simulink model "EKF_UKF_simulation"  (R2022b)
settings: Solver=VariableStepAuto  StartTime=0.0  StopTime=time  RelTol=1e-3
undefined symbols (not defined in the file): dt, R_ublox, sigbuilder_block, X_anchor, Y_anchor
libraries: sharedTrackingLibrary x2
settings Model: Creator=taha  LastModifiedBy=taha

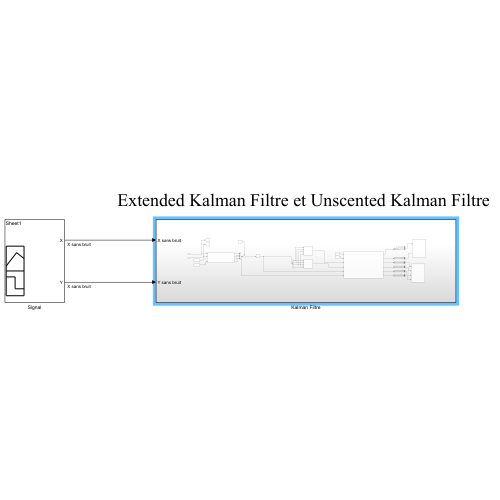
[thumbnail: Simulink's stored preview of the top-level diagram]
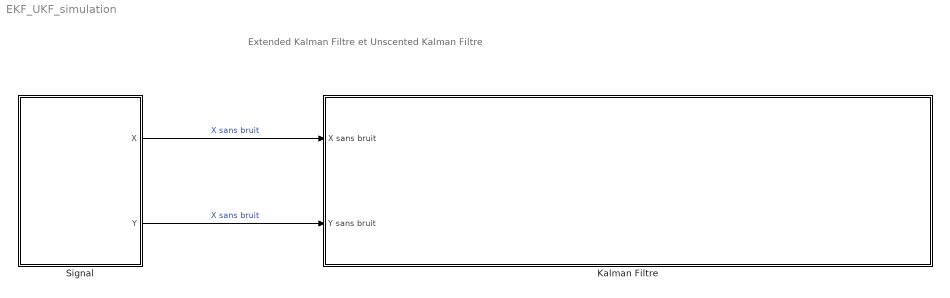
== system EKF_UKF_simulation ==
  note: Extended Kalman Filtre et Unscented Kalman Filtre
  Kalman Filtre : Subsystem
  Signal : Subsystem  Tag=STV Subsys  LoadFcn=sigbuilder_block('load');  StartFcn=sigbuilder_block('start');  StopFcn=sigbuilder_block('stop');  ClipboardFcn=sigbuilder_block('clipboard');  mask(Sigbuilder block){tuvar=[0:10]}
      mask help: Simulink:masks:SigbuilderBlock_MD
      mask init:
      | if ~strcmp(get_param(bdroot(gcbh),'SimulationStatus'),'stopped') tuvar = sigbuilder_block('maskInit'); end
      settings: CopyFcn=sigbuilder_block('copy');  DeleteFcn=sigbuilder_block('delete');  ModelCloseFcn=sigbuilder_block('modelClose');  PreSaveFcn=sigbuilder_block('preSave');  PauseFcn=sigbuilder_block('pause');  ContinueFcn=sigbuilder_block('continue');  NameChangeFcn=sigbuilder_block('namechange');  OpenFcn=sigbuilder_block('open',[6 36 1012.5 441.75 ]);  CloseFcn=sigbuilder_block('close');
      mask Display: plot(0, 0, 100, 100,[2, 2, 32, 32, 2], [68, 8, 8, 68, 68],[32, 2], [38, 38], [32, 19, 2],[53, 60, 44], [32, 17, 17, 2],[16, 16, 31, 31]);txt = getActiveGroup(gcbh);text(2, 100, txt,'verticalAlignment', 'top');
  wires:
  Signal/2(Y) -> Kalman Filtre/2(Y sans bruit)  "X sans bruit"
  Signal/1(X) -> Kalman Filtre/1(X sans bruit)  "X sans bruit"

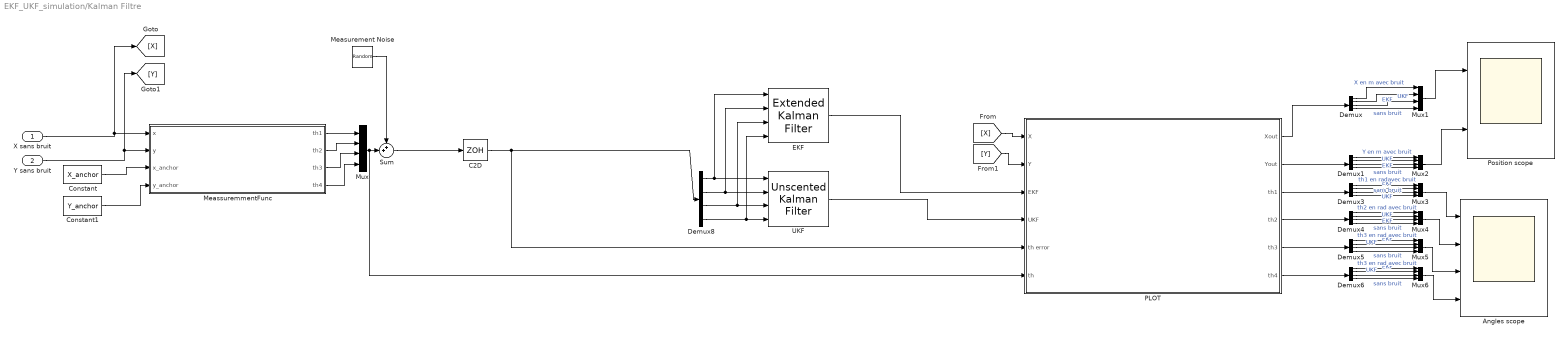
== system EKF_UKF_simulation/Kalman Filtre ==
  X sans bruit : Inport
  Y sans bruit : Inport  Port=2
  Angles scope : Scope  NumInputPorts=4
  C2D : ZeroOrderHold  SampleTime=dt
  Constant : Constant  Value=X_anchor
  Constant1 : Constant  Value=Y_anchor
  Demux{,1,3..6,8} (7 alike) : Demux
  EKF : sharedTrackingLibrary/Extended Kalman Filter  StateTransitionFcn=myStateTransitionFcn  HasStateTransitionJacobianFcn=off  HasAdditiveProcessNoise=Additive  ProcessNoise=Q  HasTimeVaryingProcessNoise=off  HasStateTransitionFcnExtraArgument=0  InitialState=x0  InitialStateCovariance=1  MeasurementFcn1=myMeasurementFcn21  HasMeasurementJacobianFcn1=off  HasMeasurementEnablePort1=off  HasAdditiveMeasurementNoise1=Additive  MeasurementNoise1=sigma_theta0  HasTimeVaryingMeasurementNoise1=off  HasMeasurementFcnExtraArgument1=0  HasMeasurementWrapping1=off  MeasurementFcn2=myMeasurementFcn22  HasMeasurementJacobianFcn2=off  HasMeasurementEnablePort2=off  HasAdditiveMeasurementNoise2=Additive  MeasurementNoise2=sigma_theta0  HasTimeVaryingMeasurementNoise2=off  HasMeasurementFcnExtraArgument2=0  HasMeasurementWrapping2=off  MeasurementFcn3=myMeasurementFcn23  HasMeasurementJacobianFcn3=off  HasMeasurementEnablePort3=off  HasAdditiveMeasurementNoise3=Additive  MeasurementNoise3=sigma_theta0  HasTimeVaryingMeasurementNoise3=off  HasMeasurementFcnExtraArgument3=0  HasMeasurementWrapping3=off  MeasurementFcn4=myMeasurementFcn24  HasMeasurementJacobianFcn4=off  HasMeasurementEnablePort4=off  HasAdditiveMeasurementNoise4=Additive  MeasurementNoise4=sigma_theta0  HasTimeVaryingMeasurementNoise4=off  HasMeasurementFcnExtraArgument4=0  HasMeasurementWrapping4=off  MeasurementFcn5=myMeasurementFcn  HasMeasurementJacobianFcn5=off  HasMeasurementEnablePort5=off  HasAdditiveMeasurementNoise5=Additive  MeasurementNoise5=1  HasTimeVaryingMeasurementNoise5=off  HasMeasurementFcnExtraArgument5=0  HasMeasurementWrapping5=off  EnableMultirate=off  StateTransitionFcnSampleTime=1  MeasurementFcn1SampleTime=1  MeasurementFcn2SampleTime=1  MeasurementFcn3SampleTime=1  MeasurementFcn4SampleTime=1  MeasurementFcn5SampleTime=1  UseCurrentEstimator=on  OutputStateCovariance=off  DataType=double  SampleTime=dt  NumberOfMeasurements=4
  MeassuremmentFunc : MATLAB Function  TreatAsAtomicUnit=on
  Measurement Noise : RandomNumber  Variance=R_ublox  SampleTime=dt
  Mux{,1..6} (7 alike) : Mux
  PLOT : Subsystem
  Position scope : Scope  NumInputPorts=2
  Sum : Sum  Inputs=++|
  UKF : sharedTrackingLibrary/Unscented Kalman Filter  StateTransitionFcn=myStateTransitionFcn  HasAdditiveProcessNoise=Additive  ProcessNoise=Q  HasTimeVaryingProcessNoise=off  HasStateTransitionFcnExtraArgument=0  InitialState=x0  InitialStateCovariance=0.1  Alpha=1  Beta=7  Kappa=3  MeasurementFcn1=myMeasurementFcn21  HasMeasurementEnablePort1=off  HasAdditiveMeasurementNoise1=Additive  MeasurementNoise1=sigma_theta0  HasTimeVaryingMeasurementNoise1=off  HasMeasurementFcnExtraArgument1=0  HasMeasurementWrapping1=off  MeasurementFcn2=myMeasurementFcn22  HasMeasurementEnablePort2=off  HasAdditiveMeasurementNoise2=Additive  MeasurementNoise2=sigma_theta0  HasTimeVaryingMeasurementNoise2=off  HasMeasurementFcnExtraArgument2=0  HasMeasurementWrapping2=off  MeasurementFcn3=myMeasurementFcn23  HasMeasurementEnablePort3=off  HasAdditiveMeasurementNoise3=Additive  MeasurementNoise3=sigma_theta0  HasTimeVaryingMeasurementNoise3=off  HasMeasurementFcnExtraArgument3=0  HasMeasurementWrapping3=off  MeasurementFcn4=myMeasurementFcn24  HasMeasurementEnablePort4=off  HasAdditiveMeasurementNoise4=Additive  MeasurementNoise4=sigma_theta0  HasTimeVaryingMeasurementNoise4=off  HasMeasurementFcnExtraArgument4=0  HasMeasurementWrapping4=off  MeasurementFcn5=myMeasurementFcn  HasMeasurementEnablePort5=off  HasAdditiveMeasurementNoise5=Additive  MeasurementNoise5=1  HasTimeVaryingMeasurementNoise5=off  HasMeasurementFcnExtraArgument5=0  HasMeasurementWrapping5=off  EnableMultirate=off  StateTransitionFcnSampleTime=1  MeasurementFcn1SampleTime=1  MeasurementFcn2SampleTime=1  MeasurementFcn3SampleTime=1  MeasurementFcn4SampleTime=1  MeasurementFcn5SampleTime=1  UseCurrentEstimator=on  OutputStateCovariance=off  DataType=double  SampleTime=dt  NumberOfMeasurements=4
  wires:
  MeassuremmentFunc/1(th1) -> Mux/1
  Measurement Noise/1 -> Sum/1
  X sans bruit/1 -> [X], MeassuremmentFunc/1(x)
  Mux/1 -> PLOT/6(th), Sum/2
  Y sans bruit/1 -> [Y], MeassuremmentFunc/2(y)
  PLOT/1(Xout) -> Demux/1
  Demux/1 -> Mux1/1  "X en m avec bruit"
  Demux/4 -> Mux1/4  "sans bruit"
  Demux/3 -> Mux1/3  "UKF"
  Demux/2 -> Mux1/2  "EKF"
  Mux1/1 -> Position scope/1
  Demux1/1 -> Mux2/1  "Y en m avec bruit"
  Demux1/4 -> Mux2/4  "sans bruit"
  Demux1/2 -> Mux2/2  "EKF"
  Demux1/3 -> Mux2/3  "UKF"
  Mux2/1 -> Position scope/2
  PLOT/2(Yout) -> Demux1/1
  MeassuremmentFunc/2(th2) -> Mux/2
  MeassuremmentFunc/3(th3) -> Mux/3
  MeassuremmentFunc/4(th4) -> Mux/4
  [X] -> PLOT/1(X)
  [Y] -> PLOT/2(Y)
  Demux4/1 -> Mux4/1  "th2 en rad avec bruit"
  Demux3/2 -> Mux3/2  "EKF"
  Demux3/3 -> Mux3/3  "UKF"
  Demux3/1 -> Mux3/1  "th1 en radavec bruit"
  Demux4/4 -> Mux4/4  "sans bruit"
  PLOT/3(th1) -> Demux3/1
  Demux4/2 -> Mux4/2  "EKF"
  Demux3/4 -> Mux3/4  "sans bruit"
  Demux4/3 -> Mux4/3  "UKF"
  PLOT/4(th2) -> Demux4/1
  Mux3/1 -> Angles scope/1
  Mux4/1 -> Angles scope/2
  Demux5/4 -> Mux5/4  "sans bruit"
  Demux5/2 -> Mux5/2  "EKF"
  Demux5/1 -> Mux5/1  "th3 en rad avec bruit"
  Mux5/1 -> Angles scope/3
  Demux5/3 -> Mux5/3  "UKF"
  PLOT/5(th3) -> Demux5/1
  Demux6/4 -> Mux6/4  "sans bruit"
  Demux6/2 -> Mux6/2  "EKF"
  Demux6/1 -> Mux6/1  "th3 en rad avec bruit"
  Demux6/3 -> Mux6/3  "UKF"
  PLOT/6(th4) -> Demux6/1
  Mux6/1 -> Angles scope/4
  Demux8/1 -> EKF/1, UKF/1
  Demux8/2 -> EKF/2, UKF/2
  Demux8/3 -> EKF/3, UKF/3
  Demux8/4 -> EKF/4, UKF/4
  Sum/1 -> C2D/1
  C2D/1 -> Demux8/1, PLOT/5(th error)
  Constant/1 -> MeassuremmentFunc/3(x_anchor)
  Constant1/1 -> MeassuremmentFunc/4(y_anchor)
  EKF/1 -> PLOT/3(EKF)
  UKF/1 -> PLOT/4(UKF)

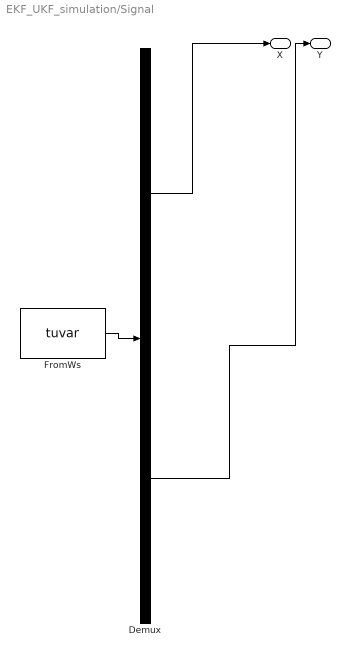
== system EKF_UKF_simulation/Signal ==
  Demux : Demux  Tag=STV Demux  Outputs=2
      settings: DisplayOption=none
  FromWs : FromWorkspace  Tag=STV FromWs  VariableName=tuvar
      SigBuilderData=|
      | common.afterFinalStr = 'Extrapolate'
      | common.sampleTime = 0
      | dataSet.timeRange = [0 9.999]
      | dataSet.name = 'Sheet1'
      | sbobj.Name = 'Signal Builder'
      | sbobj.Groups.Name = 'Sheet1'
      | sbobj.Groups.Signals(1).Name = 'X'
      | sbobj.Groups.Signals(1).XData = [0 0.001 0.002 0.003 0.004 0.005 0.006 0.007 0.008 0.009 0.01 0.011 ... (10000 elements, 1x10000)]
      | sbobj.Groups.Signals(1).YData = [2 1.99999929802 1.99999719208 1.99999368216 1.99998876824 1.9999824503 1.99997472828 1.99996560215 1.99995507184 1.99994313728 1.99992979841 1.99991505514 ... (10000 elements, 1x10000)]
      | sbobj.Groups.Signals(2).Name = 'Y'
      | sbobj.Groups.Signals(2).XData = [0 0.001 0.002 0.003 0.004 0.005 0.006 0.007 0.008 0.009 0.01 0.011 ... (10000 elements, 1x10000)]
      | sbobj.Groups.Signals(2).YData = [0 0.00251352591653 0.00502705447972 0.00754058833622 0.0100541301327 0.0125676825156 0.0150812481317 0.0175948296273 0.0201084296489 0.0226220508428 0.0251356958554 0.0276493673327 ... (10000 elements, 1x10000)]
      | sbobj.Groups.TimeRange = [0 9.999]
  X : Outport  Tag=STV Outport
  Y : Outport  Tag=STV Outport  Port=2
  wires:
  Demux/1 -> X/1
  FromWs/1 -> Demux/1
  Demux/2 -> Y/1

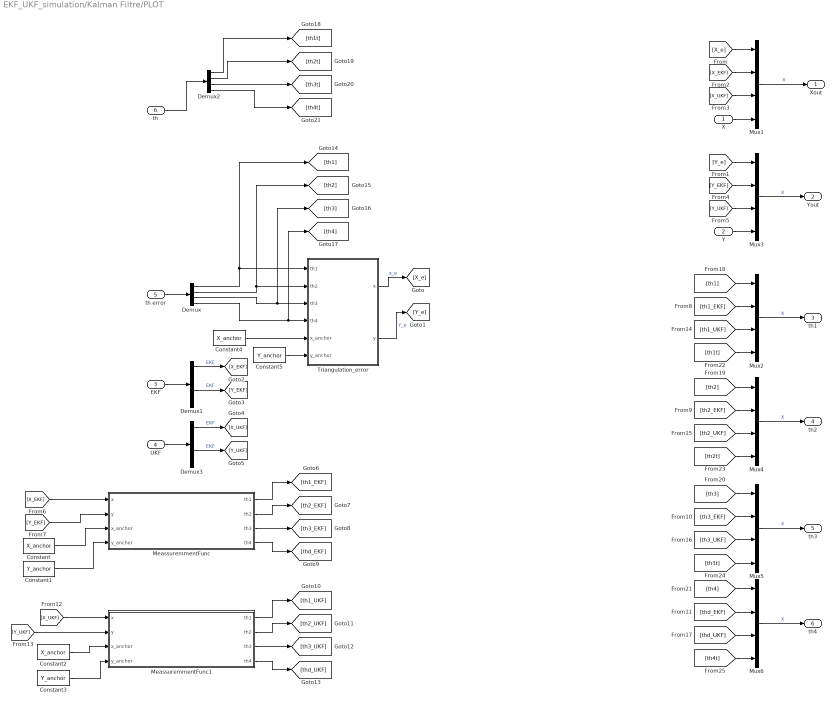
== system EKF_UKF_simulation/Kalman Filtre/PLOT ==
  X : Inport
  Y : Inport  Port=2
  EKF : Inport  Port=3
  UKF : Inport  Port=4
  th error : Inport  Port=5
  th : Inport  Port=6
  Constant : Constant  Value=X_anchor
  Constant1 : Constant  Value=Y_anchor
  Constant2 : Constant  Value=X_anchor
  Constant3 : Constant  Value=Y_anchor
  Constant4 : Constant  Value=X_anchor
  Constant5 : Constant  Value=Y_anchor
  Demux{,1..3} (4 alike) : Demux
  MeassuremmentFunc : MATLAB Function  TreatAsAtomicUnit=on
  MeassuremmentFunc1 : MATLAB Function  TreatAsAtomicUnit=on
  Mux{1..6} (6 alike) : Mux
  Triangulation_error : MATLAB Function  TreatAsAtomicUnit=on
  Xout : Outport
  Yout : Outport  Port=2
  th1 : Outport  Port=3
  th2 : Outport  Port=4
  th3 : Outport  Port=5
  th4 : Outport  Port=6
  wires:
  Mux1/1 -> Xout/1  "X"
  X/1 -> Mux1/4
  UKF/1 -> Demux3/1
  EKF/1 -> Demux1/1
  th error/1 -> Demux/1
  Demux/1 -> [th1], Triangulation_error/1(th1)
  Demux/2 -> [th2], Triangulation_error/2(th2)
  Demux/3 -> [th3], Triangulation_error/3(th3)
  Demux/4 -> [th4], Triangulation_error/4(th4)
  Triangulation_error/1(x) -> [X_e]  "x_e"
  Triangulation_error/2(y) -> [Y_e]  "Y_e"
  [X_e] -> Mux1/1
  Demux1/1 -> [X_EKF]  "EKF"
  Demux1/3 -> [Y_EKF]  "EKF"
  Demux3/1 -> [X_UKF]  "EKF"
  Demux3/3 -> [Y_UKF]  "EKF"
  [X_EKF] -> Mux1/2
  [X_UKF] -> Mux1/3
  Y/1 -> Mux3/4
  [Y_e] -> Mux3/1
  [Y_EKF] -> Mux3/2
  [Y_UKF] -> Mux3/3
  Mux3/1 -> Yout/1  "X"
  [X_EKF] -> MeassuremmentFunc/1(x)
  [Y_EKF] -> MeassuremmentFunc/2(y)
  MeassuremmentFunc/1(th1) -> [th1_EKF]
  MeassuremmentFunc/2(th2) -> [th2_EKF]
  MeassuremmentFunc/3(th3) -> [th3_EKF]
  MeassuremmentFunc/4(th4) -> [thd_EKF]
  [th1] -> Mux2/1
  [th1t] -> Mux2/4
  [th1_UKF] -> Mux2/3
  Mux2/1 -> th1/1  "X"
  [th1_EKF] -> Mux2/2
  Mux4/1 -> th2/1  "X"
  [th2_UKF] -> Mux4/3
  [th2_EKF] -> Mux4/2
  [th2t] -> Mux4/4
  [th2] -> Mux4/1
  [th3t] -> Mux5/4
  [th3_EKF] -> Mux5/2
  [th3_UKF] -> Mux5/3
  Mux5/1 -> th3/1  "X"
  [th3] -> Mux5/1
  [th4] -> Mux6/1
  Mux6/1 -> th4/1  "X"
  [thd_EKF] -> Mux6/2
  [th4t] -> Mux6/4
  [thd_UKF] -> Mux6/3
  th/1 -> Demux2/1
  Demux2/1 -> [th1t]
  Demux2/2 -> [th2t]
  Demux2/3 -> [th3t]
  Demux2/4 -> [th4t]
  Constant/1 -> MeassuremmentFunc/3(x_anchor)
  Constant1/1 -> MeassuremmentFunc/4(y_anchor)
  Constant2/1 -> MeassuremmentFunc1/3(x_anchor)
  Constant3/1 -> MeassuremmentFunc1/4(y_anchor)
  [X_UKF] -> MeassuremmentFunc1/1(x)
  [Y_UKF] -> MeassuremmentFunc1/2(y)
  MeassuremmentFunc1/1(th1) -> [th1_UKF]
  MeassuremmentFunc1/2(th2) -> [th2_UKF]
  MeassuremmentFunc1/3(th3) -> [th3_UKF]
  MeassuremmentFunc1/4(th4) -> [thd_UKF]
  Constant4/1 -> Triangulation_error/5(x_anchor)
  Constant5/1 -> Triangulation_error/6(y_anchor)

== matlab function EKF_UKF_simulation/Kalman Filtre/MeassuremmentFunc ==
  data: x input; th1 output; y input; th2 output; th3 output; th4 output; x_anchor input; y_anchor input
function [th1,th2,th3, th4] = meassuremmentFunc(x,y,x_anchor,y_anchor)
th1=atan2(y,x);
th2=atan2(y,x-x_anchor);
th3=atan2(y-y_anchor,x-x_anchor);
th4=atan2(y-y_anchor,x);

== matlab function EKF_UKF_simulation/Kalman Filtre/PLOT/MeassuremmentFunc ==
  data: x input; th1 output; y input; th2 output; th3 output; th4 output; x_anchor input; y_anchor input
function [th1,th2,th3, th4] = meassuremmentFunc(x,y,x_anchor,y_anchor)
th1=atan2(y,x);
th2=atan2(y,x-x_anchor);
th3=atan2(y-y_anchor,x-x_anchor);
th4=atan2(y-y_anchor,x);

== matlab function EKF_UKF_simulation/Kalman Filtre/PLOT/Triangulation_error ==
  data: x output; th1 input; y output; th2 input; th3 input; th4 input; x_anchor input; y_anchor input
function [x, y] = Triangulation(th1,th2,th3,th4,x_anchor,y_anchor)
    % angles: list of angles between point A and each reference point
    % ref_points: list of reference points with known coordinates (x_i, y_i)
    angles=[th1 th2 th3 th4];
    ref_points = [0 0 ; x_anchor 0 ; x_anchor y_anchor ; 0 y_anchor];
    N = 4;
    A = [0 0 ; 0 0 ; 0 0 ; 0 0 ];
    b = [0;0;0;0];
    for i = 1:N
        angle = angles(i);
        x_i = ref_points(i, 1);
        y_i = ref_points(i, 2);
        A(i, :) = [sin(angle), -cos(angle)];
        b(i) = sin(angle)*x_i - cos(angle)*y_i;
    end
    
    AA = inv(A' * A);
    BB = A' * b;
    X = AA * BB;
    x = X(1);
    y = X(2);

== matlab function EKF_UKF_simulation/Kalman Filtre/PLOT/MeassuremmentFunc1 ==
  data: x input; th1 output; y input; th2 output; th3 output; th4 output; x_anchor input; y_anchor input
function [th1,th2,th3, th4] = meassuremmentFunc(x,y,x_anchor,y_anchor)
th1=atan2(y,x);
th2=atan2(y,x-x_anchor);
th3=atan2(y-y_anchor,x-x_anchor);
th4=atan2(y-y_anchor,x);
